simulink model "ControlPID"  (R2020a)
settings: Solver=FixedStepDiscrete  StartTime=0.0  StopTime=10.0  RelTol=1e-3
model workspace (MAT data in the model file):
  Kd = Simulink.Parameter
  Kd.Value = 0.0008954
  Kd.DataType = 'double'
  Kd.Dimensions = [1 1]
  Ki = Simulink.Parameter
  Ki.Value = 0.39
  Ki.DataType = 'double'
  Ki.Dimensions = [1 1]
  Kp = Simulink.Parameter
  Kp.Value = 0.0121
  Kp.DataType = 'double'
  Kp.Dimensions = [1 1]
  Ts = Simulink.Parameter
  Ts.Value = 0.01
  Ts.DataType = 'double'
  Ts.Dimensions = [1 1]
undefined symbols (not defined in the file): DiscIntNeverNeededParam
libraries: GPIO_Lib x3, TIMERS_Lib x2, USART_Lib x1, simulink x1, STM32_Config_Lib x1
settings Model: OrderedModelArguments=off  Creator=Lenovo  LastModifiedBy=Lenovo
settings OptimizationCC: DefaultParameterBehavior=Inlined  EnhancedBackFolding=on  PassReuseOutputArgsAs=Individual arguments  ZeroExternalMemoryAtStartup=off  ZeroInternalMemoryAtStartup=off  OptimizeBlockOrder=speed  DifferentSizesBufferReuse=on  OptimizationCustomize=off  EfficientTunableParamExpr=on
settings DebuggingCC: MultiTaskDSMMsg=none  ParameterTunabilityLossMsg=error
settings HardwareCC: ProdBitPerPointer=32  ProdBitPerSizeT=32  ProdBitPerPtrDiffT=32  ProdLargestAtomicInteger=Long  ProdWordSize=32  ProdHWDeviceType=STM32CortexM
settings SFSimCC: MATLABDynamicMemAlloc=off
settings RTWCC: Description=stm32 (Embedded Target)  SystemTargetFile=stm32.tlc  TemplateMakefile=stm32.tmf  GenerateReport=on
settings CodeAppCC: ForceParamTrailComments=on  IgnoreCustomStorageClasses=off  MaxIdLength=64  OperatorAnnotations=on  SimulinkDataObjDesc=on  SFDataObjDesc=on  CustomSymbolStrType=$N$R$M  SimulinkBlockComments=off
settings STFCustomTargetCC: TargetLangStandard=C99 (ISO)  CodeReplacementLibrary=ARM CMSIS SIN COS  MultiwordLength=256  ParMdlRefBuildCompliant=on  IncludeMdlTerminateFcn=off  CombineOutputUpdateFcns=on  ERTCustomFileBanners=on  SupportContinuousTime=off  SupportNonInlinedSFcns=off  RemoveResetFunc=on  MATLABClassNameForMDSCustomization=Simulink.SoftwareTarget.ERTCustomization  SystemTargetFile=stm32.tlc
settings ERTTargetCC: TargetLangStandard=C99 (ISO)  CodeReplacementLibrary=ARM CMSIS SIN COS  CompOptLevelCompliant=off  ConcurrentExecutionCompliant=off  IncludeMdlTerminateFcn=off  ModelStepFunctionPrototypeControlCompliant=off  CPPClassGenCompliant=off  UseToolchainInfoCompliant=off  ExtModeStaticAllocSize=256  ExtModeMexFile=ext_serial_win32_comm  ExtModeMexArgs=0,1,115200,10  InlinedParameterPlacement=NonHierarchical  ERTSrcFileBannerTemplate=sourceFileTemplate.cgt  ERTHdrFileBannerTemplate=sourceFileTemplate.cgt  ERTDataSrcFileTemplate=sourceFileTemplate.cgt  ERTDataHdrFileTemplate=sourceFileTemplate.cgt  ERTCustomFileTemplate=customRoutineProcess.tlc

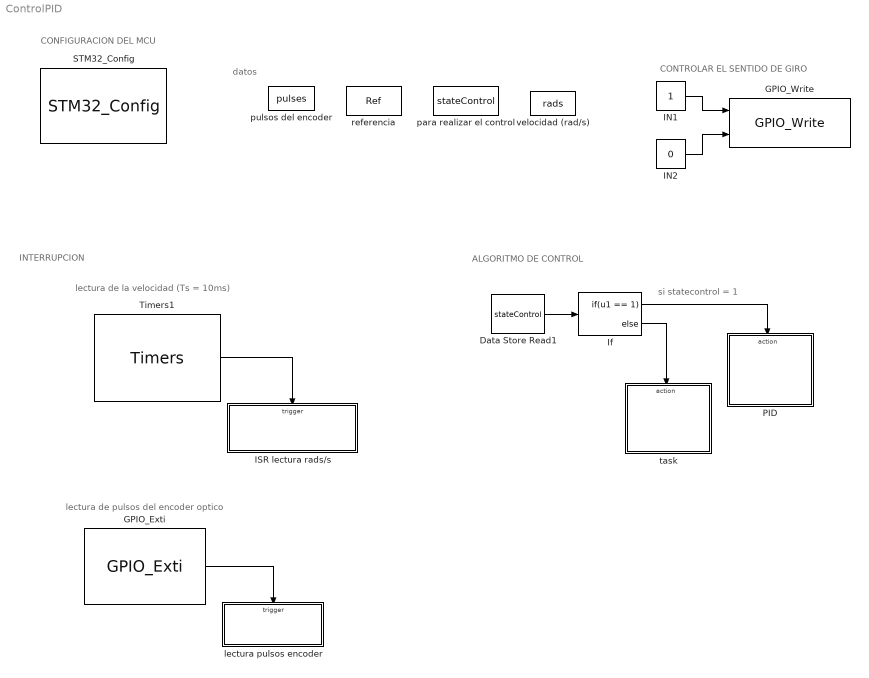
== system ControlPID ==
  note: si statecontrol = 1
  note: INTERRUPCION
  note: ALGORITMO DE CONTROL
  note: lectura de la velocidad (Ts = 10ms)
  note: lectura de pulsos del encoder optico
  note: CONFIGURACION DEL MCU
  note: CONTROLAR EL SENTIDO DE GIRO
  note: datos
  Data Store Read1 : DataStoreRead  DataStoreName=stateControl
  GPIO_Exti : GPIO_Lib/GPIO_Exti  Port_name=GPIOA  Pin_0=on  Pin_1=off  Pin_2=off  Pin_3=off  Pin_4=off  Pin_5=off  Pin_6=off  Pin_7=off  Pin_8=off  Pin_9=off  Pin_10=off  Pin_11=off  Pin_12=off  Pin_13=off  Pin_14=off  Pin_15=off  PinList=GPIOA0
      settings: SourceProductName=Target Support Package - STM32 Adapter
  GPIO_Write : GPIO_Lib/GPIO_Write  Port_name=GPIOB  Pin0=off  Toggle_Pin0=off  Pin1=on  Toggle_Pin1=off  Pin2=off  Toggle_Pin2=off  Pin3=off  Toggle_Pin3=off  Pin4=off  Toggle_Pin4=off  Pin5=off  Toggle_Pin5=off  Pin6=on  Toggle_Pin6=off  Pin7=off  Toggle_Pin7=off  Pin8=off  Toggle_Pin8=off  Pin9=off  Toggle_Pin9=off  Pin10=off  Toggle_Pin10=off  Pin11=off  Toggle_Pin11=off  Pin12=off  Toggle_Pin12=off  Pin13=off  Toggle_Pin13=off  Pin14=off  Toggle_Pin14=off  Pin15=off  Toggle_Pin15=off  PinList="GPIOB1  3  6"
      settings: SourceProductName=Target Support Package - STM32 Adapter
  IN1 : Constant
  IN2 : Constant  Value=0
  ISR lectura rads/s : Subsystem  TreatAsAtomicUnit=on
  If : If  IfExpression=u1 == 1
  PID : Subsystem  TreatAsAtomicUnit=on
  STM32_Config : STM32_Config_Lib/STM32_Config  Priority=0  Project_Path=.\  Config_File=ControlPID.ioc  MCU_Name=STM32L412KBUx
      settings: SourceProductName=Target Support Package - STM32 Adapter
  Timers1 : TIMERS_Lib/Timers  currentTIM=TIM6  TIM_Name=TIM6  sysUsingTimer=off  TIM_APBClock=80000000  TIM_Set_Clk=off  TIM_Prescaler=79  TIM_Clock=1000000.00  Variable_frequency=off  TIM_Set_OutFreq=off  TIM_ARR=10000-1  Output_frequency=100.01  Repetition_counter=0  TIM_Mode=Up  TIM_DMA=none  TIM_IRQ=off  TIM_IRQ_ONLY=on  TIM_UP=on  TIM_TRG=off  TIM_COM=off  TIM_BRK=off  NbTIM=2  CH1_enable=off  CH1N_enable=off  CH1_type=Unknown  CH1_DMA=off  CH1_int=off  CH1_edge=Rising  CH1_div=1  CH1_variable_duty=off  CH1_set_pulse=off  CH1_output_duty=0.00  CH1_pulse=0  CH2_enable=off  CH2N_enable=off  CH2_type=Unknown  CH2_DMA=off  CH2_int=off  CH2_edge=Rising  CH2_div=1  CH2_variable_duty=off  CH2_set_pulse=off  CH2_output_duty=0.00  CH2_pulse=0  CH3_enable=off  CH3N_enable=off  CH3_type=Unknown  CH3_DMA=off  CH3_int=off  CH3_edge=Rising  CH3_div=1  CH3_variable_duty=off  CH3_set_pulse=off  CH3_output_duty=0.00  CH3_pulse=0  CH4_enable=off  CH4N_enable=off  CH4_type=Unknown  CH4_DMA=off  CH4_int=off  CH4_edge=Rising  CH4_div=1  CH4_variable_duty=off  CH4_set_pulse=off  CH4_output_duty=0.00  CH4_pulse=0
      settings: SourceProductName=Target Support Package - STM32 Adapter
  "lectura pulsos encoder " : Subsystem  TreatAsAtomicUnit=on
  para realizar el control : DataStoreMemory  DataStoreName=stateControl  ReadBeforeWriteMsg=warning  WriteAfterWriteMsg=warning  WriteAfterReadMsg=warning  ShowAdditionalParam=off
  pulsos del encoder : DataStoreMemory  DataStoreName=pulses  ReadBeforeWriteMsg=warning  WriteAfterWriteMsg=warning  WriteAfterReadMsg=warning  ShowAdditionalParam=off
  referencia : DataStoreMemory  DataStoreName=Ref  ReadBeforeWriteMsg=warning  WriteAfterWriteMsg=warning  WriteAfterReadMsg=warning  ShowAdditionalParam=off
  task : Subsystem  TreatAsAtomicUnit=on
  velocidad (rad/s) : DataStoreMemory  DataStoreName=rads  ReadBeforeWriteMsg=warning  WriteAfterWriteMsg=warning  WriteAfterReadMsg=warning  ShowAdditionalParam=off
  wires:
  Timers1/1 -> ISR lectura rads/s/Trigger
  IN2/1 -> GPIO_Write/2
  IN1/1 -> GPIO_Write/1
  GPIO_Exti/1 -> "lectura pulsos encoder "/Trigger
  Data Store Read1/1 -> If/1
  If/1 -> PID/Action
  If/2 -> task/Action

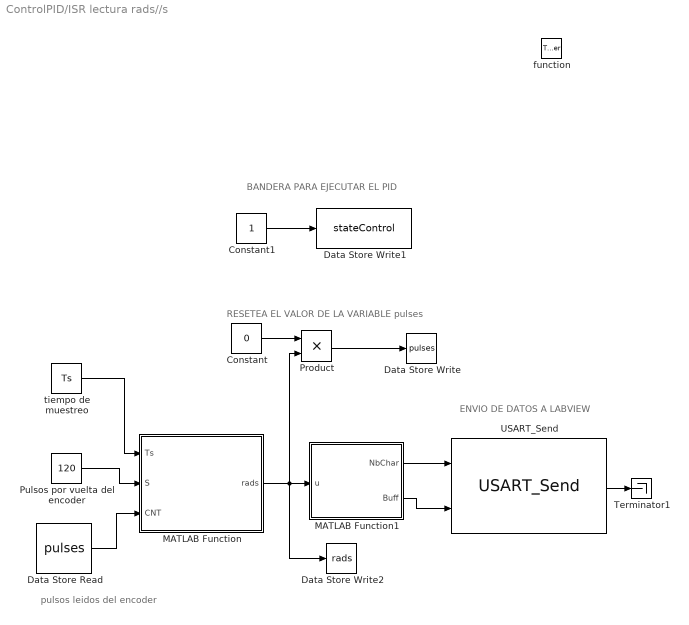
== system ControlPID/ISR lectura rads//s ==
  note: pulsos leidos del encoder
  note: BANDERA PARA EJECUTAR EL PID
  note: RESETEA EL VALOR DE LA VARIABLE pulses
  note: ENVIO DE DATOS A LABVIEW
  function : TriggerPort  TriggerType=function-call  VariantControl=Variant
  Constant : Constant  Value=0
  Constant1 : Constant
  Data Store Read : DataStoreRead  DataStoreName=pulses
  Data Store Write : DataStoreWrite  DataStoreName=pulses
  Data Store Write1 : DataStoreWrite  DataStoreName=stateControl
  Data Store Write2 : DataStoreWrite  DataStoreName=rads
  MATLAB Function : MATLAB Function  TreatAsAtomicUnit=on
  MATLAB Function1 : MATLAB Function  TreatAsAtomicUnit=on
  Product : Product
  Pulsos por vuelta del encoder : Constant  Value=120
  Terminator1 : Terminator
  USART_Send : USART_Lib/USART_Send  USART_name=USART2  Buff_size=512  nbUsart=1  usartMode=Asynchronous  usartDma_Rx=off  usartDma_Tx=off  usartIt=on
      settings: SourceProductName=Target Support Package - STM32 Adapter
  tiempo de muestreo : Constant  Value=Ts
  wires:
  Data Store Read/1 -> MATLAB Function/3(CNT)
  Pulsos por vuelta del encoder/1 -> MATLAB Function/2(S)
  tiempo de muestreo/1 -> MATLAB Function/1(Ts)
  MATLAB Function/1(rads) -> Data Store Write2/1, Product/2, MATLAB Function1/1(u)
  MATLAB Function1/2(Buff) -> USART_Send/2
  MATLAB Function1/1(NbChar) -> USART_Send/1
  USART_Send/1 -> Terminator1/1
  Constant/1 -> Product/1
  Product/1 -> Data Store Write/1
  Constant1/1 -> Data Store Write1/1

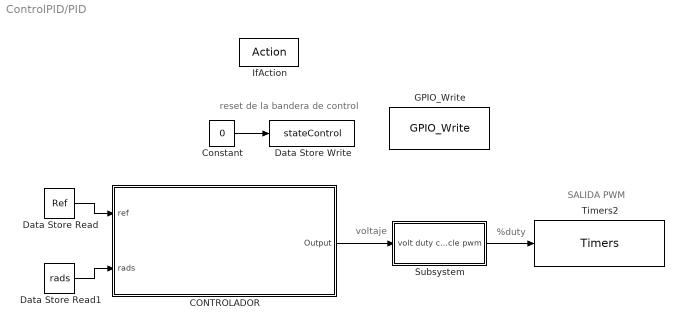
== system ControlPID/PID ==
  note: SALIDA PWM
  note: reset de la bandera de control
  note: %duty
  note: voltaje
  IfAction : ActionPort  ActionPortLabel=if(u1 == 1)
  CONTROLADOR : Subsystem
  Constant : Constant  Value=0
  Data Store Read : DataStoreRead  DataStoreName=Ref
  Data Store Read1 : DataStoreRead  DataStoreName=rads
  Data Store Write : DataStoreWrite  DataStoreName=stateControl
  GPIO_Write : GPIO_Lib/GPIO_Write  Port_name=GPIOB  Pin0=off  Toggle_Pin0=off  Pin1=off  Toggle_Pin1=off  Pin2=off  Toggle_Pin2=off  Pin3=on  Toggle_Pin3=on  Pin4=off  Toggle_Pin4=off  Pin5=off  Toggle_Pin5=off  Pin6=off  Toggle_Pin6=off  Pin7=off  Toggle_Pin7=off  Pin8=off  Toggle_Pin8=off  Pin9=off  Toggle_Pin9=off  Pin10=off  Toggle_Pin10=off  Pin11=off  Toggle_Pin11=off  Pin12=off  Toggle_Pin12=off  Pin13=off  Toggle_Pin13=off  Pin14=off  Toggle_Pin14=off  Pin15=off  Toggle_Pin15=off  PinList="GPIOB1  3  6"
      settings: SourceProductName=Target Support Package - STM32 Adapter
  Subsystem : Subsystem
  Timers2 : TIMERS_Lib/Timers  currentTIM=TIM15  TIM_Name=TIM15  sysUsingTimer=off  TIM_APBClock=80000000  TIM_Set_Clk=off  TIM_Prescaler=40-1  TIM_Clock=2000000.00  Variable_frequency=off  TIM_Set_OutFreq=off  TIM_ARR=50  Output_frequency=40000.00  Repetition_counter=0  TIM_Mode=Up  TIM_DMA=none  TIM_IRQ=off  TIM_IRQ_ONLY=on  TIM_UP=off  TIM_TRG=off  TIM_COM=off  TIM_BRK=off  NbTIM=2  CH1_enable=off  CH1N_enable=off  CH1_type=Unknown  CH1_DMA=off  CH1_int=off  CH1_edge=Rising  CH1_div=1  CH1_variable_duty=off  CH1_set_pulse=off  CH1_output_duty=0.00  CH1_pulse=0  CH2_enable=on  CH2N_enable=off  CH2_type=Output_PWM  CH2_DMA=off  CH2_int=off  CH2_edge=Rising  CH2_div=1  CH2_variable_duty=on  CH2_set_pulse=off  CH2_output_duty=0.00  CH2_pulse=0  CH3_enable=off  CH3N_enable=off  CH3_type=Unknown  CH3_DMA=off  CH3_int=off  CH3_edge=Rising  CH3_div=1  CH3_variable_duty=off  CH3_set_pulse=off  CH3_output_duty=0.00  CH3_pulse=0  CH4_enable=off  CH4N_enable=off  CH4_type=Unknown  CH4_DMA=off  CH4_int=off  CH4_edge=Rising  CH4_div=1  CH4_variable_duty=off  CH4_set_pulse=off  CH4_output_duty=0.00  CH4_pulse=0
      settings: SourceProductName=Target Support Package - STM32 Adapter
  wires:
  Data Store Read/1 -> CONTROLADOR/1(ref)
  Constant/1 -> Data Store Write/1
  Data Store Read1/1 -> CONTROLADOR/2(rads)
  CONTROLADOR/1(Output) -> Subsystem/1(volt)
  Subsystem/1(duty cycle pwm) -> Timers2/1

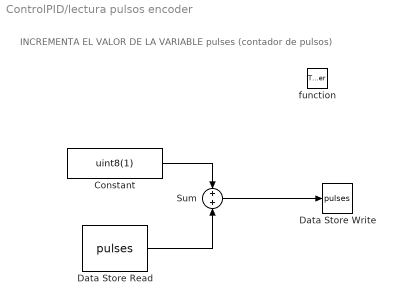
== system ControlPID/lectura pulsos encoder  ==
  note: INCREMENTA EL VALOR DE LA VARIABLE pulses (contador de pulsos)
  function : TriggerPort  TriggerType=function-call  VariantControl=Variant
  Constant : Constant  Value=uint8(1)
  Data Store Read : DataStoreRead  DataStoreName=pulses
  Data Store Write : DataStoreWrite  DataStoreName=pulses
  Sum : Sum
  wires:
  Constant/1 -> Sum/1
  Data Store Read/1 -> Sum/2
  Sum/1 -> Data Store Write/1

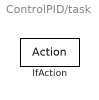
== system ControlPID/task ==
  IfAction : ActionPort  ActionPortLabel=else

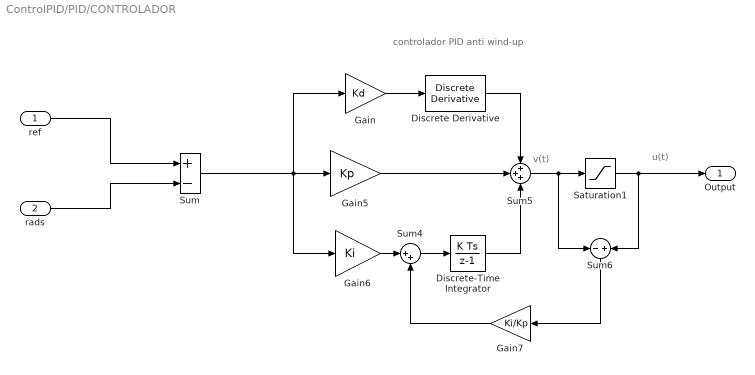
== system ControlPID/PID/CONTROLADOR ==
  note: v(t)
  note: controlador PID anti wind-up
  note: u(t)
  ref : Inport
  rads : Inport  Port=2
  Discrete Derivative : simulink/Discrete/Discrete Derivative  gainval=Kd  ICPrevScaledInput=0.0  OutMin=[]  OutMax=[]  OutDataType=fixdt(1, 16)  OutScaling=2^-10  DoSatur=off
  Discrete-Time Integrator : DiscreteIntegrator  gainval=1  SampleTime=Ts  ICPrevOutput=DiscIntNeverNeededParam  ICPrevScaledInput=DiscIntNeverNeededParam
  Gain : Gain  Gain=Kd
  Gain5 : Gain  Gain=Kp
  Gain6 : Gain  Gain=Ki
  Gain7 : Gain  Gain=Ki/Kp
  Saturation1 : Saturate  UpperLimit=8.37  LowerLimit=0
  Sum : Sum  Inputs=+-
  Sum4 : Sum  Inputs=|++
  Sum5 : Sum  Inputs=+++
  Sum6 : Sum  Inputs=-+
  Output : Outport
  wires:
  Sum4/1 -> Discrete-Time Integrator/1
  Sum/1 -> Gain/1, Gain6/1, Gain5/1
  Discrete-Time Integrator/1 -> Sum5/3
  Gain7/1 -> Sum4/2
  Sum6/1 -> Gain7/1
  Gain5/1 -> Sum5/2
  Saturation1/1 -> Output/1, Sum6/2
  Gain6/1 -> Sum4/1
  Discrete Derivative/1 -> Sum5/1
  Sum5/1 -> Sum6/1, Saturation1/1
  ref/1 -> Sum/1
  rads/1 -> Sum/2
  Gain/1 -> Discrete Derivative/1

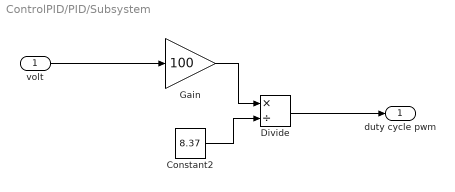
== system ControlPID/PID/Subsystem ==
  volt : Inport
  Constant2 : Constant  Value=8.37
  Divide : Product  Inputs=*/
  Gain : Gain  Gain=100
  duty cycle pwm : Outport
  wires:
  Constant2/1 -> Divide/2
  Gain/1 -> Divide/1
  volt/1 -> Gain/1
  Divide/1 -> duty cycle pwm/1

== matlab function ControlPID/ISR lectura rads//s/MATLAB Function1 ==
  data: u input; NbChar output; Buff output
function [NbChar, Buff] = convert(u)
if coder.target('Sfun')
    %executing in Matlab, Buff is null
    Buff = uint32(0);
    NbChar = uint16(0);
else
    %executing in the generated code
    buffer = zeros(1,15,'uint8');
%     coder.ceval('sprintf',coder.wref(buffer),['%2.2f',0],u);
%     tmp = uint8(' rad/s');
%     y = [buffer(1:4),tmp,13,10,0];
%     Buff = coder.ceval('getBuffPtr',coder.ref(y));
%     NbChar = uint16(size(y,2));
%     y = [buffer(1:4),13,10,0];
%     Buff = coder.ceval('getBuffPtr',coder.ref(buffer));
%     NbChar = uint16(size(y,2));
    Buff = coder.ceval('getBuffPtr',coder.ref(buffer));
    NbChar = coder.ceval('sprintf',coder.wref(buffer),['%.2f\r\n',0],u);
end

== matlab function ControlPID/ISR lectura rads//s/MATLAB Function ==
  data: Ts input; rads output; S input; CNT input
function rads = calc_rads(Ts, S, CNT)
if coder.target('Sfun')
    %executing in Matlab, Buff is null
    rads = double(0);
else
    rpm = CNT * 60.0 / (Ts * S);
    rads = rpm * (2 * pi) / 60;
end
